simulink model "Demo_veDYNA_cs"  (Simulink 7.6)
settings: Solver=ode1  StartTime=0  StopTime=15  FixedStep=1/500  RelTol=1e-3
PreLoadFcn:
  | PreScanveDYNAPreLoadFcn(bdroot);
  | check_NUTS_defined;
  | 
  | assignin('base',['model_closed_' bdroot],false);
PostLoadFcn:
  | PreScanveDYNAPostLoadFcn(bdroot);
  | 
InitFcn:
  | vdy_SetExternalInputSource('ManLongCtrl',1,'Brake','other');
  | vdy_SetExternalInputSource('ManLongCtrl',1,'EngineTorque','other');
  | vdy_SetExternalInputSource('ManLatCtrl',1,'Steering','other');
  | 
  | PreScanveDYNAInitFcn(bdroot);
  | PreScanExperimentInitFcn(bdroot)
StopFcn:
  | PreScanExperimentStopFcn(bdroot)
undefined symbols (not defined in the file): at_period, CPT, vm_at_pulsewidth, vm_driver_dflt_gain, x_ini_VRML, y_ini_VRML, z_ini_VRML
libraries: dyna_cpt_lib x93, simulink x16, simulink_extras x14, PreScanSimulinkLibrary x6, anilib x3, dyna_lib x3, dyna_manctrl_lib x2, dyna_road_lib x2, PreScanUsefulBlocks x1, dyna_io_lib x1, dyna_demo_lib x1, dyna_usr_maneuver_states_lib x1
(part 5 of 8)

== system Demo_veDYNA_cs/Mazda_RX8_1/Simple ACC/Engine Torque Control/Demux Vehicle Info ==
  Vehicle Info : Inport
  vSoll : Inport  Port=2
  Bus Selector : BusSelector  OutputSignals=EngineTorqueMax[Nm],EngineTorqueMin[Nm],VehicleSpeed[m|s],TyreRadiusStatFront[m],GearRatioFront[],TyreRadiusStatRear[m],GearRatioRear[],VehicleMass[kg],EngineInertia[kgm2]
  gear_ratio : Subsystem
  mmot diff : Subsystem
  theta_red : Subsystem
  mmot_MAX : Outport
  mmot_MIN : Outport  Port=2
  v_akt1 : Outport  Port=3
  mmot_diff : Outport  Port=4
  wires:
  vSoll/1 -> mmot diff/5(vSoll)
  mmot diff/1(Out1) -> mmot_diff/1
  Bus Selector/2 -> mmot_MIN/1  "<EngineTorqueMin[Nm]>"
  Bus Selector/1 -> mmot_MAX/1  "<EngineTorqueMax[Nm]>"
  Bus Selector/3 -> v_akt1/1, mmot diff/1(vIst)  "<VehicleSpeed[m|s]>"
  theta_red/1(Theta) -> mmot diff/3(Theta)
  gear_ratio/1(GearRatio) -> theta_red/1(gear ratio), mmot diff/2(gear_ratio)
  Vehicle Info/1 -> Bus Selector/1
  Bus Selector/4 -> gear_ratio/1(RStatF)  "<TyreRadiusStatFront[m]>"
  Bus Selector/5 -> gear_ratio/2(GearRatioF)  "<GearRatioFront[]>"
  Bus Selector/6 -> gear_ratio/3(RStatR)  "<TyreRadiusStatRear[m]>"
  Bus Selector/7 -> gear_ratio/4(GearRatioR)  "<GearRatioRear[]>"
  Bus Selector/8 -> theta_red/2(VehMass)  "<VehicleMass[kg]>"
  Bus Selector/9 -> mmot diff/4(Theta Mot)  "<EngineInertia[kgm2]>"

== system Demo_veDYNA_cs/Mazda_RX8_1/Simple ACC/Engine Torque Control/Distance Control ==
  mmot_MAX : Inport
  mmot_MIN : Inport  Port=2
  v_akt : Inport  Port=3
  s_diff : Inport  Port=4
  Constant1 : Constant  Value=0
  Data Type Conversion1 : DataTypeConversion  SaturateOnIntegerOverflow=on  RndMeth=Zero
  Gain3 : Gain  Gain=-.1  SaturateOnIntegerOverflow=on  OutDataTypeStr=Inherit: Same as input  ParamDataTypeStr=Inherit: Same as input
  MinMax1 : MinMax  Function=max  Inputs=2  SaturateOnIntegerOverflow=on  InputSameDT=on
  MinMax2 : MinMax  Inputs=2  SaturateOnIntegerOverflow=on  InputSameDT=on
  P-Controller : Gain  Gain=6
  Product1 : Product  SaturateOnIntegerOverflow=on  InputSameDT=on  OutDataTypeStr=Inherit: Same as first input
  Relational Operator1 : RelationalOperator  Operator=>  InputSameDT=on
  Saturation1 : Saturate  UpperLimit=100  LowerLimit=0
  Sum : Sum  Inputs=|+-  SaturateOnIntegerOverflow=on  InputSameDT=on  OutDataTypeStr=Inherit: Same as first input
  dist_ratio : Gain  Gain=1.2  SaturateOnIntegerOverflow=on  OutDataTypeStr=Inherit: Same as input  ParamDataTypeStr=Inherit: Same as input
  Engine Torque : Outport
  Brake Pedal : Outport  Port=2
  wires:
  Saturation1/1 -> Brake Pedal/1
  Product1/1 -> Saturation1/1
  Gain3/1 -> Product1/2
  Data Type Conversion1/1 -> Product1/1
  Relational Operator1/1 -> Data Type Conversion1/1
  Constant1/1 -> Relational Operator1/1
  P-Controller/1 -> Gain3/1, Relational Operator1/2, MinMax1/1
  MinMax2/1 -> Engine Torque/1
  MinMax1/1 -> MinMax2/2
  mmot_MAX/1 -> MinMax2/1
  mmot_MIN/1 -> MinMax1/2
  dist_ratio/1 -> Sum/2
  Sum/1 -> P-Controller/1
  v_akt/1 -> dist_ratio/1
  s_diff/1 -> Sum/1

== system Demo_veDYNA_cs/Mazda_RX8_1/Simple ACC/Engine Torque Control/Speed Control ==
  mmot_MAX : Inport
  mmot_MIN : Inport  Port=2
  mmot_diff : Inport  Port=3
  MinMax : MinMax  Function=max  Inputs=2  SaturateOnIntegerOverflow=on  InputSameDT=on
  MinMax1 : MinMax  Inputs=2  SaturateOnIntegerOverflow=on  InputSameDT=on
  P-Controller : Gain  Gain=6
  Engine Torque : Outport
  wires:
  mmot_MIN/1 -> MinMax/2
  mmot_MAX/1 -> MinMax1/1
  MinMax1/1 -> Engine Torque/1
  MinMax/1 -> MinMax1/2
  P-Controller/1 -> MinMax/1
  mmot_diff/1 -> P-Controller/1

== system Demo_veDYNA_cs/Nissan_Cabstar_1/SELF_Demux/compas converter/cart2compas ==
  Angle [deg] : Inport
  Constant : Constant  Value=90
  Constant1 : Constant  Value=360
  Gain : Gain  Gain=1/360
  Gain1 : Gain  Gain=360
  Gain2 : Gain  Gain=-1
  Rounding Function : Rounding
  Sum : Sum  Inputs=|-+
  Sum1 : Sum  Inputs=-+|
  Sum2 : Sum  Inputs=++|
  heading [deg] : Outport
  wires:
  Sum2/1 -> heading [deg]/1
  Constant1/1 -> Sum2/1
  Gain2/1 -> Sum2/2
  Constant/1 -> Sum1/1
  Sum1/1 -> Sum/2, Gain/1
  Sum/1 -> Gain2/1
  Angle [deg]/1 -> Sum1/2
  Gain1/1 -> Sum/1
  Rounding Function/1 -> Gain1/1
  Gain/1 -> Rounding Function/1

== system Demo_veDYNA_cs/Nissan_Cabstar_1/Trajectories/Traj2State1/Traj2State2 ==
  traj : Inport
  MuxState : Subsystem
  Traj2MuxState_Ext : Subsystem
  state : Outport
  wires:
  Traj2MuxState_Ext/9(Y [rad]) -> MuxState/9(Y [rad])
  Traj2MuxState_Ext/8(P [rad]) -> MuxState/8(P [rad])
  Traj2MuxState_Ext/7(R [rad]) -> MuxState/7(R [rad])
  Traj2MuxState_Ext/6(dz [m/s]) -> MuxState/6(dz [m/s])
  Traj2MuxState_Ext/5(dy [m/s]) -> MuxState/5(dy [m/s])
  Traj2MuxState_Ext/4(dx [m/s]) -> MuxState/4(dx [m/s])
  Traj2MuxState_Ext/3(z [m]) -> MuxState/3(z [m])
  Traj2MuxState_Ext/2(y [m]) -> MuxState/2(y [m])
  Traj2MuxState_Ext/1(x [m]) -> MuxState/1(x [m])
  MuxState/1(state) -> state/1
  traj/1 -> Traj2MuxState_Ext/1(Traj)

== system Demo_veDYNA_cs/STATE_BMW_X5_1/state2FullState/limit roll/Substitute 90 & 270 deg (and its plurals) ==
  Angle [rad] : Inport
  270 deg detection : simulink/Model Verification/Check  Static Gap  Description=u <= 269.5 || 270.5 <= u  SystemSampleTime=-1  max=270.5  max_included=on  min=269.5  min_included=on  enabled=on  stopWhenAssertionFail=off  export=on  icon=graphic
  90 deg detection : simulink/Model Verification/Check  Static Gap  Description=u <= 89.5 || 90.5 <= u  SystemSampleTime=-1  max=90.5  max_included=on  min=89.5  min_included=on  enabled=on  stopWhenAssertionFail=off  export=on  icon=graphic
  Angle 0-360 deg limiter : Subsystem
  Degrees to Radians : simulink_extras/Transformations/Degrees to Radians  SystemSampleTime=-1
  Radians to Degrees : simulink_extras/Transformations/Radians to Degrees  SystemSampleTime=-1
  Substitution  Value : Constant  Value=269.5
  Substitution Value : Constant  Value=89.5
  Switch : Switch  Threshold=0.5
  Switch1 : Switch  Threshold=0.5
  Subst Angle [rad] : Outport
  wires:
  Angle [rad]/1 -> Radians to Degrees/1
  Degrees to Radians/1 -> Subst Angle [rad]/1
  Radians to Degrees/1 -> Angle 0-360 deg limiter/1(Angle [deg])
  Switch1/1 -> Degrees to Radians/1
  Substitution  Value/1 -> Switch1/3
  270 deg detection/1 -> Switch1/2
  Switch/1 -> Switch1/1, 270 deg detection/1
  Substitution Value/1 -> Switch/3
  90 deg detection/1 -> Switch/2
  Angle 0-360 deg limiter/1(LimAngle [deg]) -> 90 deg detection/1, Switch/1

== system Demo_veDYNA_cs/STATE_Mazda_RX8_1/state2FullState/limit roll/Substitute 90 & 270 deg (and its plurals) ==
  Angle [rad] : Inport
  270 deg detection : simulink/Model Verification/Check  Static Gap  Description=u <= 269.5 || 270.5 <= u  SystemSampleTime=-1  max=270.5  max_included=on  min=269.5  min_included=on  enabled=on  stopWhenAssertionFail=off  export=on  icon=graphic
  90 deg detection : simulink/Model Verification/Check  Static Gap  Description=u <= 89.5 || 90.5 <= u  SystemSampleTime=-1  max=90.5  max_included=on  min=89.5  min_included=on  enabled=on  stopWhenAssertionFail=off  export=on  icon=graphic
  Angle 0-360 deg limiter : Subsystem
  Degrees to Radians : simulink_extras/Transformations/Degrees to Radians  SystemSampleTime=-1
  Radians to Degrees : simulink_extras/Transformations/Radians to Degrees  SystemSampleTime=-1
  Substitution  Value : Constant  Value=269.5
  Substitution Value : Constant  Value=89.5
  Switch : Switch  Threshold=0.5
  Switch1 : Switch  Threshold=0.5
  Subst Angle [rad] : Outport
  wires:
  Angle [rad]/1 -> Radians to Degrees/1
  Degrees to Radians/1 -> Subst Angle [rad]/1
  Radians to Degrees/1 -> Angle 0-360 deg limiter/1(Angle [deg])
  Switch1/1 -> Degrees to Radians/1
  Substitution  Value/1 -> Switch1/3
  270 deg detection/1 -> Switch1/2
  Switch/1 -> Switch1/1, 270 deg detection/1
  Substitution Value/1 -> Switch/3
  90 deg detection/1 -> Switch/2
  Angle 0-360 deg limiter/1(LimAngle [deg]) -> 90 deg detection/1, Switch/1

== system Demo_veDYNA_cs/STATE_Nissan_Cabstar_1/state2FullState/limit roll/Substitute 90 & 270 deg (and its plurals) ==
  Angle [rad] : Inport
  270 deg detection : simulink/Model Verification/Check  Static Gap  Description=u <= 269.5 || 270.5 <= u  SystemSampleTime=-1  max=270.5  max_included=on  min=269.5  min_included=on  enabled=on  stopWhenAssertionFail=off  export=on  icon=graphic
  90 deg detection : simulink/Model Verification/Check  Static Gap  Description=u <= 89.5 || 90.5 <= u  SystemSampleTime=-1  max=90.5  max_included=on  min=89.5  min_included=on  enabled=on  stopWhenAssertionFail=off  export=on  icon=graphic
  Angle 0-360 deg limiter : Subsystem
  Degrees to Radians : simulink_extras/Transformations/Degrees to Radians  SystemSampleTime=-1
  Radians to Degrees : simulink_extras/Transformations/Radians to Degrees  SystemSampleTime=-1
  Substitution  Value : Constant  Value=269.5
  Substitution Value : Constant  Value=89.5
  Switch : Switch  Threshold=0.5
  Switch1 : Switch  Threshold=0.5
  Subst Angle [rad] : Outport
  wires:
  Angle [rad]/1 -> Radians to Degrees/1
  Degrees to Radians/1 -> Subst Angle [rad]/1
  Radians to Degrees/1 -> Angle 0-360 deg limiter/1(Angle [deg])
  Switch1/1 -> Degrees to Radians/1
  Substitution  Value/1 -> Switch1/3
  270 deg detection/1 -> Switch1/2
  Switch/1 -> Switch1/1, 270 deg detection/1
  Substitution Value/1 -> Switch/3
  90 deg detection/1 -> Switch/2
  Angle 0-360 deg limiter/1(LimAngle [deg]) -> 90 deg detection/1, Switch/1

== system Demo_veDYNA_cs/Vedyna_Vehicle/CPT_MDL/MDL_PAR/BrkHyd ==
  System Instance 1 : Subsystem
      mask Display: disp('[Generated]')

== system Demo_veDYNA_cs/Vedyna_Vehicle/CPT_MDL/MDL_PAR/ClutchCtrl ==
  System Instance 1 : Subsystem
      mask Display: disp('[Generated]')

== system Demo_veDYNA_cs/Vedyna_Vehicle/CPT_MDL/MDL_PAR/Contact ==
  System Instance 1 : Subsystem
      mask Display: disp('[Generated]')
  System Instance 2 : Subsystem
      mask Display: disp('[Generated]')
  System Instance 3 : Subsystem
      mask Display: disp('[Generated]')
  System Instance 4 : Subsystem
      mask Display: disp('[Generated]')
  System Instance 5 : Subsystem
      mask Display: disp('[Generated]')
  System Instance 6 : Subsystem
      mask Display: disp('[Generated]')
  System Instance 7 : Subsystem
      mask Display: disp('[Generated]')
  System Instance 8 : Subsystem
      mask Display: disp('[Generated]')

== system Demo_veDYNA_cs/Vedyna_Vehicle/CPT_MDL/MDL_PAR/Driver ==
  System Instance 1 : Subsystem
      mask Display: disp('[Generated]')

== system Demo_veDYNA_cs/Vedyna_Vehicle/CPT_MDL/MDL_PAR/Engine ==
  System Instance 1 : Subsystem
      mask Display: disp('[Generated]')

== system Demo_veDYNA_cs/Vedyna_Vehicle/CPT_MDL/MDL_PAR/GearCtrl ==
  System Instance 1 : Subsystem
      mask Display: disp('[Generated]')

== system Demo_veDYNA_cs/Vedyna_Vehicle/CPT_MDL/MDL_PAR/ManLatCtrl ==
  System Instance 1 : Subsystem
      mask Display: disp('[Generated]')

== system Demo_veDYNA_cs/Vedyna_Vehicle/CPT_MDL/MDL_PAR/ManLongCtrl ==
  System Instance 1 : Subsystem
      mask Display: disp('[Generated]')

== system Demo_veDYNA_cs/Vedyna_Vehicle/CPT_MDL/MDL_PAR/ManSchedule ==

== system Demo_veDYNA_cs/Vedyna_Vehicle/CPT_MDL/MDL_PAR/Tmeasy ==
  System Instance 1 : Subsystem
      mask Display: disp('[Generated]')
  System Instance 2 : Subsystem
      mask Display: disp('[Generated]')
  System Instance 3 : Subsystem
      mask Display: disp('[Generated]')
  System Instance 4 : Subsystem
      mask Display: disp('[Generated]')
  System Instance 5 : Subsystem
      mask Display: disp('[Generated]')
  System Instance 6 : Subsystem
      mask Display: disp('[Generated]')
  System Instance 7 : Subsystem
      mask Display: disp('[Generated]')
  System Instance 8 : Subsystem
      mask Display: disp('[Generated]')

== system Demo_veDYNA_cs/Vedyna_Vehicle/CPT_MDL/MDL_PAR/Wheel ==
  System Instance 1 : Subsystem
      mask Display: disp('[Generated]')
  System Instance 2 : Subsystem
      mask Display: disp('[Generated]')
  System Instance 3 : Subsystem
      mask Display: disp('[Generated]')
  System Instance 4 : Subsystem
      mask Display: disp('[Generated]')
  System Instance 5 : Subsystem
      mask Display: disp('[Generated]')
  System Instance 6 : Subsystem
      mask Display: disp('[Generated]')
  System Instance 7 : Subsystem
      mask Display: disp('[Generated]')
  System Instance 8 : Subsystem
      mask Display: disp('[Generated]')

== system Demo_veDYNA_cs/Vedyna_Vehicle/CPT_MDL/MDL_SW/BrkHyd ==
  System Instance 1 : Subsystem
      mask Display: disp('[Generated]')

== system Demo_veDYNA_cs/Vedyna_Vehicle/CPT_MDL/MDL_SW/Chassis ==
  System Instance 1 : Subsystem
      mask Display: disp('[Generated]')

== system Demo_veDYNA_cs/Vedyna_Vehicle/CPT_MDL/MDL_SW/ClutchCtrl ==
  System Instance 1 : Subsystem
      mask Display: disp('[Generated]')

== system Demo_veDYNA_cs/Vedyna_Vehicle/CPT_MDL/MDL_SW/Contact ==
  System Instance 1 : Subsystem
      mask Display: disp('[Generated]')
  System Instance 2 : Subsystem
      mask Display: disp('[Generated]')
  System Instance 3 : Subsystem
      mask Display: disp('[Generated]')
  System Instance 4 : Subsystem
      mask Display: disp('[Generated]')
  System Instance 5 : Subsystem
      mask Display: disp('[Generated]')
  System Instance 6 : Subsystem
      mask Display: disp('[Generated]')
  System Instance 7 : Subsystem
      mask Display: disp('[Generated]')
  System Instance 8 : Subsystem
      mask Display: disp('[Generated]')

== system Demo_veDYNA_cs/Vedyna_Vehicle/CPT_MDL/MDL_SW/Driveline ==
  System Instance 1 : Subsystem
      mask Display: disp('[Generated]')

== system Demo_veDYNA_cs/Vedyna_Vehicle/CPT_MDL/MDL_SW/Driver ==
  System Instance 1 : Subsystem
      mask Display: disp('[Generated]')

== system Demo_veDYNA_cs/Vedyna_Vehicle/CPT_MDL/MDL_SW/Engine ==
  System Instance 1 : Subsystem
      mask Display: disp('[Generated]')

== system Demo_veDYNA_cs/Vedyna_Vehicle/CPT_MDL/MDL_SW/GearCtrl ==
  System Instance 1 : Subsystem
      mask Display: disp('[Generated]')

== system Demo_veDYNA_cs/Vedyna_Vehicle/CPT_MDL/MDL_SW/ManLatCtrl ==
  System Instance 1 : Subsystem
      mask Display: disp('[Generated]')

== system Demo_veDYNA_cs/Vedyna_Vehicle/CPT_MDL/MDL_SW/ManLongCtrl ==
  System Instance 1 : Subsystem
      mask Display: disp('[Generated]')

== system Demo_veDYNA_cs/Vedyna_Vehicle/CPT_MDL/MDL_SW/ManSchedule ==
  System Instance 1 : Subsystem
      mask Display: disp('[Generated]')
  System Instance 2 : Subsystem
      mask Display: disp('[Generated]')
  System Instance 3 : Subsystem
      mask Display: disp('[Generated]')

== system Demo_veDYNA_cs/Vedyna_Vehicle/CPT_MDL/MDL_SW/Road ==
  System Instance 1 : Subsystem
      mask Display: disp('[Generated]')

== system Demo_veDYNA_cs/Vedyna_Vehicle/CPT_MDL/MDL_SW/Simctrl ==
  System Instance 1 : Subsystem
      mask Display: disp('[Generated]')

== system Demo_veDYNA_cs/Vedyna_Vehicle/CPT_MDL/MDL_SW/Tmeasy ==
  System Instance 1 : Subsystem
      mask Display: disp('[Generated]')
  System Instance 2 : Subsystem
      mask Display: disp('[Generated]')
  System Instance 3 : Subsystem
      mask Display: disp('[Generated]')
  System Instance 4 : Subsystem
      mask Display: disp('[Generated]')
  System Instance 5 : Subsystem
      mask Display: disp('[Generated]')
  System Instance 6 : Subsystem
      mask Display: disp('[Generated]')
  System Instance 7 : Subsystem
      mask Display: disp('[Generated]')
  System Instance 8 : Subsystem
      mask Display: disp('[Generated]')

== system Demo_veDYNA_cs/Vedyna_Vehicle/CPT_MDL/MDL_SW/Vehicle ==
  System Instance 1 : Subsystem
      mask Display: disp('[Generated]')

== system Demo_veDYNA_cs/Vedyna_Vehicle/CPT_MDL/MDL_SW/Wheel ==
  System Instance 1 : Subsystem
      mask Display: disp('[Generated]')
  System Instance 2 : Subsystem
      mask Display: disp('[Generated]')
  System Instance 3 : Subsystem
      mask Display: disp('[Generated]')
  System Instance 4 : Subsystem
      mask Display: disp('[Generated]')
  System Instance 5 : Subsystem
      mask Display: disp('[Generated]')
  System Instance 6 : Subsystem
      mask Display: disp('[Generated]')
  System Instance 7 : Subsystem
      mask Display: disp('[Generated]')
  System Instance 8 : Subsystem
      mask Display: disp('[Generated]')

== system Demo_veDYNA_cs/Vedyna_Vehicle/vdy_mdl/Maneuver Control/HCI Switch Driver ==
  Mux3 : Mux  Inputs=3
  SW_ClutchCtrl_1_HCI : dyna_cpt_lib/CPT_MDL_HCI_SW_ACCESS  Tag=vedynaCPT_MDL_HCI_SW_ACCESS  component=ClutchCtrl  system_inst=1  parameter=HCI
  SW_Driver_1_HCI : dyna_cpt_lib/CPT_MDL_HCI_SW_ACCESS  Tag=vedynaCPT_MDL_HCI_SW_ACCESS  component=Driver  system_inst=1  parameter=HCI
  SW_GearCtrl_1_HCI : dyna_cpt_lib/CPT_MDL_HCI_SW_ACCESS  Tag=vedynaCPT_MDL_HCI_SW_ACCESS  component=GearCtrl  system_inst=1  parameter=HCI
  HCI manCtrl : Outport
  wires:
  Mux3/1 -> HCI manCtrl/1
  SW_ClutchCtrl_1_HCI/1 -> Mux3/3
  SW_GearCtrl_1_HCI/1 -> Mux3/2
  SW_Driver_1_HCI/1 -> Mux3/1

== system Demo_veDYNA_cs/Vedyna_Vehicle/vdy_mdl/Maneuver Control/HCI Switches ==
  Mux : Mux  Inputs=3
  SW_ManSchedule_1_HCI : dyna_cpt_lib/CPT_MDL_HCI_SW_ACCESS  Tag=vedynaCPT_MDL_HCI_SW_ACCESS  component=ManSchedule  system_inst=1  parameter=HCI
  SW_ManSchedule_2_HCI : dyna_cpt_lib/CPT_MDL_HCI_SW_ACCESS  Tag=vedynaCPT_MDL_HCI_SW_ACCESS  component=ManSchedule  system_inst=2  parameter=HCI
  SW_ManSchedule_3_HCI : dyna_cpt_lib/CPT_MDL_HCI_SW_ACCESS  Tag=vedynaCPT_MDL_HCI_SW_ACCESS  component=ManSchedule  system_inst=3  parameter=HCI
  "HCI Switches " : Outport
  wires:
  SW_ManSchedule_3_HCI/1 -> Mux/3
  SW_ManSchedule_2_HCI/1 -> Mux/2
  SW_ManSchedule_1_HCI/1 -> Mux/1
  Mux/1 -> "HCI Switches "/1

== system Demo_veDYNA_cs/Vedyna_Vehicle/vdy_mdl/Maneuver Control/Maneuver Controller Inputs ==
  Clutch Control Inputs : Subsystem
  Driver Inputs : Subsystem
  Gear Control Inputs : Subsystem
  Lateral Control Inputs : Subsystem
  Longitudinal Control Inputs : Subsystem
  "Longitudinal Control Inputs " : Outport
  "Lateral Control Inputs " : Outport  Port=2
  "Driver Inputs " : Outport  Port=3
  "Gear Control Inputs " : Outport  Port=4
  "Clutch Control Inputs " : Outport  Port=5
  wires:
  Driver Inputs/1(Driver Inputs) -> "Driver Inputs "/1
  Gear Control Inputs/1(Gear Control Inputs) -> "Gear Control Inputs "/1
  Clutch Control Inputs/1(Clutch Control Inputs) -> "Clutch Control Inputs "/1
  Lateral Control Inputs/1(Lateral Control Inputs) -> "Lateral Control Inputs "/1
  Longitudinal Control Inputs/1(Longitudinal Control Inputs) -> "Longitudinal Control Inputs "/1

== system Demo_veDYNA_cs/Vedyna_Vehicle/vdy_mdl/Maneuver Control/Maneuver Scheduler Inputs ==
  Vehicle Info : Inport
  Demux : Demux  Outputs=[2,-1]
  Demux1 : Demux  Outputs=[3 1 1 1 1]
  Dot Product : DotProduct  InputSameDT=on  OutDataTypeStr=Inherit: Inherit via internal rule
  Math Functio : Math  Operator=sqrt  SaturateOnIntegerOverflow=on
  Mux1 : Mux  Inputs=3
  Mux2 : Mux  Inputs=6
  Road Information : dyna_road_lib/Road Information  comp_name=Road  RdQueryTyp=xy  nq=1  rd_info_lib=vm_road_info_lib
  Selector4 : Selector  InputPortWidth=21  IndexOptions=Index vector (dialog)  Indices=[1]  OutputSizes=1
  User Definition of Maneuver End States : dyna_usr_maneuver_states_lib/User Definition of Maneuver End States
  m/s_km/h : Gain  Gain=3.6  SaturateOnIntegerOverflow=on  OutDataTypeStr=Inherit: Same as input  ParamDataTypeStr=Inherit: Same as input
  rad_deg : Gain  Gain=180/pi  SaturateOnIntegerOverflow=on  OutDataTypeStr=Inherit: Same as input  ParamDataTypeStr=Inherit: Same as input
  rad_deg1 : Gain  Gain=1e-5  SaturateOnIntegerOverflow=on  OutDataTypeStr=Inherit: Same as input  ParamDataTypeStr=Inherit: Same as input
  rad_deg2 : Gain  Gain=180/pi  SaturateOnIntegerOverflow=on  OutDataTypeStr=Inherit: Same as input  ParamDataTypeStr=Inherit: Same as input
  state_from_vehicleinfo : Selector  IndexOptions=Index vector (dialog)  Indices=[7,8,10,11,12,38,14,66,65]  OutputSizes=1
  Control States : Outport
  wires:
  Demux1/1 -> Dot Product/2, Dot Product/1  "velocity[m/s]"
  Math Functio/1 -> m/s_km/h/1
  Dot Product/1 -> Math Functio/1
  User Definition of Maneuver End States/1 -> Mux2/6
  Mux2/1 -> Mux1/3
  Demux/2 -> Demux1/1
  rad_deg2/1 -> Mux2/5  "[deg/s]"
  rad_deg1/1 -> Mux2/4  "[bar]"
  rad_deg/1 -> Mux2/2  "[deg]"
  m/s_km/h/1 -> Mux2/1  "[km/h]"
  Demux1/5 -> rad_deg2/1  "roll rate [rad/s]"
  Demux1/2 -> rad_deg/1  "steering wheel angle [rad]"
  Demux1/3 -> Mux2/3  "lateral acc.[m/s**2]"
  Demux1/4 -> rad_deg1/1  "brake pressure [Pa]"
  state_from_vehicleinfo/1 -> Demux/1
  Demux/1 -> Road Information/1
  Selector4/1 -> Mux1/2  "distance [m]"
  Mux1/1 -> Control States/1
  [vdy_Simctrl_tsim] -> Mux1/1  "Simulation time [s]"
  Road Information/1 -> Selector4/1
  Vehicle Info/1 -> state_from_vehicleinfo/1

== system Demo_veDYNA_cs/Vedyna_Vehicle/vdy_mdl/Road/veDYNA Road Subsystem ==
  note: veDYNA Road Subsystem
  note: COPYRIGHT 2002 by TESIS DYNAware GmbH
  SyncIn : Inport
  HCI Switch : Subsystem
  veDYNA Road : dyna_road_lib/veDYNA Road
  SyncOut : Outport
  wires:
  HCI Switch/1(HCI Switch) -> veDYNA Road/2
  veDYNA Road/1 -> SyncOut/1
  SyncIn/1 -> veDYNA Road/1

== system Demo_veDYNA_cs/Vedyna_Vehicle/vdy_mdl/Simulation Control/veDYNA Simulation Control Subsystem ==
  note: veDYNA Simulation Control Subsystem
  note: COPYRIGHT 2002 by TESIS DYNAware GmbH
  SyncIn : Inport
  SW_Simctrl_1_Reset : dyna_cpt_lib/CPT_MDL_SW_ACCESS  Tag=vedynaCPT_MDL_HCI_ACCESS  component=Simctrl  system_inst=1  parameter=Reset
  veDYNA Simulation Control : dyna_simctrl_lib/veDYNA Simulation Control  Tag=vedynaSimctrlMask
  SyncOut : Outport
  wires:
  SW_Simctrl_1_Reset/1 -> veDYNA Simulation Control/2
  veDYNA Simulation Control/1 -> SyncOut/1
  SyncIn/1 -> veDYNA Simulation Control/1

== system Demo_veDYNA_cs/Vedyna_Vehicle/vdy_mdl/Vehicle System/veDYNA Vehicle Subsystem ==
  note: veDYNA Vehicle Subsystem
  note: COPYRIGHT 2002 by TESIS DYNAware GmbH
  SyncIn : Inport
  Maneuver Commands : Inport  Port=2
  Input from I/O : Inport  Port=3
  External Body Forces : Inport  Port=4
  Brake System : Subsystem
  External Vehicle Inputs (from I/O) : Subsystem
  HCI Switches : Subsystem
  Maneuver Commands Splitter : Subsystem
  Mux : Mux  Inputs=2
  Selector : Selector  InputPortWidth=32  IndexOptions=Index vector (dialog)  Indices=[1:4]  OutputSizes=1
  Selector1 : Selector  InputPortWidth=32  IndexOptions=Index vector (dialog)  Indices=[5:18]  OutputSizes=1
  Vehicle Outputs to I/O : Subsystem
  veDYNA Vehicle : dyna_vehicle_lib/veDYNA Vehicle
  Output to I/O : Outport
  Vehicle Info : Outport  Port=2
  Reference System : Outport  Port=3
  SyncOut : Outport  Port=4
  wires:
  HCI Switches/1(HCI Switches) -> veDYNA Vehicle/7
  Selector1/1 -> Brake System/2(I/O Vector)
  Selector/1 -> External Vehicle Inputs (from I/O)/2(I/O Vector)
  Input from I/O/1 -> Selector/1, Selector1/1
  Mux/1 -> Vehicle Info/1
  Vehicle Outputs to I/O/2(SyncOut) -> SyncOut/1
  Vehicle Outputs to I/O/1(Output to IO) -> Output to I/O/1
  veDYNA Vehicle/3 -> Vehicle Outputs to I/O/1(SyncIn)
  External Vehicle Inputs (from I/O)/2(External Inputs) -> veDYNA Vehicle/5
  External Body Forces/1 -> veDYNA Vehicle/6
  External Vehicle Inputs (from I/O)/1(SyncOut) -> Brake System/1(SyncIn)
  veDYNA Vehicle/1 -> Mux/2
  Brake System/1(Brake Hydraulics Info) -> Mux/1
  Brake System/2(SyncOut) -> veDYNA Vehicle/1
  Brake System/3(Master Cylinder Pressure) -> veDYNA Vehicle/2
  Brake System/4(Wheel Cylinder Pressures) -> veDYNA Vehicle/3
  veDYNA Vehicle/2 -> Reference System/1
  Maneuver Commands Splitter/4(Maneuver Commands to Vehicle) -> veDYNA Vehicle/4
  Maneuver Commands/1 -> Maneuver Commands Splitter/2(Maneuver Commands)
  SyncIn/1 -> Maneuver Commands Splitter/1(SyncIn)
  Maneuver Commands Splitter/3(Maneuver Commands to Brake System) -> Brake System/3(Brake Pedal Position)
  Maneuver Commands Splitter/2(Maneuver Commands to External Inputs) -> External Vehicle Inputs (from I/O)/3(Maneuver Commands)
  Maneuver Commands Splitter/1(SyncOut) -> External Vehicle Inputs (from I/O)/1(SyncIn)

== system Demo_veDYNA_cs/BMW_X5_1/Trajectories/Traj2State1/Traj2State2/MuxState ==
  x [m] : Inport
  y [m] : Inport  Port=2
  z [m] : Inport  Port=3
  dx [m/s] : Inport  Port=4
  dy [m/s] : Inport  Port=5
  dz [m/s] : Inport  Port=6
  R [rad] : Inport  Port=7
  P [rad] : Inport  Port=8
  Y [rad] : Inport  Port=9
  Mux : Mux  Inputs=9
  state : Outport
  wires:
  z [m]/1 -> Mux/3
  y [m]/1 -> Mux/2
  x [m]/1 -> Mux/1
  Y [rad]/1 -> Mux/9
  P [rad]/1 -> Mux/8
  R [rad]/1 -> Mux/7
  dz [m/s]/1 -> Mux/6
  dy [m/s]/1 -> Mux/5
  dx [m/s]/1 -> Mux/4
  Mux/1 -> state/1

== system Demo_veDYNA_cs/BMW_X5_1/Trajectories/Traj2State1/Traj2State2/Traj2MuxState_Ext ==
  Traj : Inport
  Terminator{1..9} (9 alike) : Terminator
  demux : Subsystem
  x [m] : Outport
  y [m] : Outport  Port=2
  z [m] : Outport  Port=3
  dx [m/s] : Outport  Port=4
  dy [m/s] : Outport  Port=5
  dz [m/s] : Outport  Port=6
  R [rad] : Outport  Port=7
  P [rad] : Outport  Port=8
  Y [rad] : Outport  Port=9
  wires:
  demux/9(Y) -> Y [rad]/1
  demux/7(R) -> R [rad]/1
  demux/5(vely) -> dy [m/s]/1
  demux/4(velx) -> dx [m/s]/1
  demux/10(velR) -> Terminator4/1
  demux/11(velP) -> Terminator5/1
  demux/12(velY) -> Terminator1/1
  demux/13(accx) -> Terminator8/1
  demux/14(accy) -> Terminator9/1
  demux/15(accz) -> Terminator7/1
  demux/18(accY) -> Terminator2/1
  demux/16(accR) -> Terminator3/1
  demux/17(accP) -> Terminator6/1
  demux/3(z) -> z [m]/1
  Traj/1 -> demux/1(traj)
  demux/6(velz) -> dz [m/s]/1
  demux/1(x) -> x [m]/1
  demux/2(y) -> y [m]/1
  demux/8(P) -> P [rad]/1

== system Demo_veDYNA_cs/Mazda_RX8_1/Simple ACC/Engine Torque Control/Demux Vehicle Info/gear_ratio ==
  RStatF : Inport
  GearRatioF : Inport  Port=2
  RStatR : Inport  Port=3
  GearRatioR : Inport  Port=4
  Product1 : Product  Inputs=/*  SaturateOnIntegerOverflow=on  InputSameDT=on  OutDataTypeStr=Inherit: Same as first input
  Product2 : Product  Inputs=/*  SaturateOnIntegerOverflow=on  InputSameDT=on  OutDataTypeStr=Inherit: Same as first input
  Sum : Sum  Inputs=|++  SaturateOnIntegerOverflow=on  InputSameDT=on  OutDataTypeStr=Inherit: Same as first input
  GearRatio : Outport
  wires:
  Sum/1 -> GearRatio/1
  Product2/1 -> Sum/1
  Product1/1 -> Sum/2
  RStatF/1 -> Product2/1
  GearRatioF/1 -> Product2/2
  RStatR/1 -> Product1/1
  GearRatioR/1 -> Product1/2

== system Demo_veDYNA_cs/Mazda_RX8_1/Simple ACC/Engine Torque Control/Demux Vehicle Info/mmot diff ==
  vIst : Inport
  gear_ratio : Inport  Port=2
  Theta : Inport  Port=3
  Theta Mot : Inport  Port=4
  vSoll : Inport  Port=5
  Product : Product  Inputs=3  SaturateOnIntegerOverflow=on  InputSameDT=on  OutDataTypeStr=Inherit: Same as first input
  Sum : Sum  Inputs=|++  SaturateOnIntegerOverflow=on  InputSameDT=on  OutDataTypeStr=Inherit: Same as first input
  Sum1 : Sum  Inputs=+-  SaturateOnIntegerOverflow=on  InputSameDT=on  OutDataTypeStr=Inherit: Same as first input
  Out1 : Outport
  wires:
  Product/1 -> Out1/1
  Sum1/1 -> Product/1
  Sum/1 -> Product/3
  gear_ratio/1 -> Product/2
  vSoll/1 -> Sum1/1
  vIst/1 -> Sum1/2
  Theta/1 -> Sum/1
  Theta Mot/1 -> Sum/2

== system Demo_veDYNA_cs/Mazda_RX8_1/Simple ACC/Engine Torque Control/Demux Vehicle Info/theta_red ==
  gear ratio : Inport
  VehMass : Inport  Port=2
  Constant : Constant
  Math Function : Math  Operator=square  SaturateOnIntegerOverflow=on
  Product1 : Product  Inputs=/*  SaturateOnIntegerOverflow=on  InputSameDT=on  OutDataTypeStr=Inherit: Same as first input
  Sum : Sum  Inputs=++|  SaturateOnIntegerOverflow=on  InputSameDT=on  OutDataTypeStr=Inherit: Same as first input
  Theta : Outport
  wires:
  Constant/1 -> Sum/1
  Sum/1 -> Product1/1
  Math Function/1 -> Sum/2
  gear ratio/1 -> Math Function/1
  Product1/1 -> Theta/1
  VehMass/1 -> Product1/2

== system Demo_veDYNA_cs/Nissan_Cabstar_1/Trajectories/Traj2State1/Traj2State2/MuxState ==
  x [m] : Inport
  y [m] : Inport  Port=2
  z [m] : Inport  Port=3
  dx [m/s] : Inport  Port=4
  dy [m/s] : Inport  Port=5
  dz [m/s] : Inport  Port=6
  R [rad] : Inport  Port=7
  P [rad] : Inport  Port=8
  Y [rad] : Inport  Port=9
  Mux : Mux  Inputs=9
  state : Outport
  wires:
  z [m]/1 -> Mux/3
  y [m]/1 -> Mux/2
  x [m]/1 -> Mux/1
  Y [rad]/1 -> Mux/9
  P [rad]/1 -> Mux/8
  R [rad]/1 -> Mux/7
  dz [m/s]/1 -> Mux/6
  dy [m/s]/1 -> Mux/5
  dx [m/s]/1 -> Mux/4
  Mux/1 -> state/1

== system Demo_veDYNA_cs/Nissan_Cabstar_1/Trajectories/Traj2State1/Traj2State2/Traj2MuxState_Ext ==
  Traj : Inport
  Terminator{1..9} (9 alike) : Terminator
  demux : Subsystem
  x [m] : Outport
  y [m] : Outport  Port=2
  z [m] : Outport  Port=3
  dx [m/s] : Outport  Port=4
  dy [m/s] : Outport  Port=5
  dz [m/s] : Outport  Port=6
  R [rad] : Outport  Port=7
  P [rad] : Outport  Port=8
  Y [rad] : Outport  Port=9
  wires:
  demux/9(Y) -> Y [rad]/1
  demux/7(R) -> R [rad]/1
  demux/5(vely) -> dy [m/s]/1
  demux/4(velx) -> dx [m/s]/1
  demux/10(velR) -> Terminator4/1
  demux/11(velP) -> Terminator5/1
  demux/12(velY) -> Terminator1/1
  demux/13(accx) -> Terminator8/1
  demux/14(accy) -> Terminator9/1
  demux/15(accz) -> Terminator7/1
  demux/18(accY) -> Terminator2/1
  demux/16(accR) -> Terminator3/1
  demux/17(accP) -> Terminator6/1
  demux/3(z) -> z [m]/1
  Traj/1 -> demux/1(traj)
  demux/6(velz) -> dz [m/s]/1
  demux/1(x) -> x [m]/1
  demux/2(y) -> y [m]/1
  demux/8(P) -> P [rad]/1

== system Demo_veDYNA_cs/STATE_BMW_X5_1/state2FullState/limit roll/Substitute 90 & 270 deg (and its plurals)/Angle 0-360 deg limiter ==
  Angle [deg] : Inport
  Gain : Gain  Gain=1/360
  Gain1 : Gain  Gain=360
  Rounding Function : Rounding
  Sum : Sum  Inputs=|-+
  LimAngle [deg] : Outport
  wires:
  Gain/1 -> Rounding Function/1
  Rounding Function/1 -> Gain1/1
  Gain1/1 -> Sum/1
  Angle [deg]/1 -> Gain/1, Sum/2
  Sum/1 -> LimAngle [deg]/1

== system Demo_veDYNA_cs/STATE_Mazda_RX8_1/state2FullState/limit roll/Substitute 90 & 270 deg (and its plurals)/Angle 0-360 deg limiter ==
  Angle [deg] : Inport
  Gain : Gain  Gain=1/360
  Gain1 : Gain  Gain=360
  Rounding Function : Rounding
  Sum : Sum  Inputs=|-+
  LimAngle [deg] : Outport
  wires:
  Gain/1 -> Rounding Function/1
  Rounding Function/1 -> Gain1/1
  Gain1/1 -> Sum/1
  Angle [deg]/1 -> Gain/1, Sum/2
  Sum/1 -> LimAngle [deg]/1

== system Demo_veDYNA_cs/STATE_Nissan_Cabstar_1/state2FullState/limit roll/Substitute 90 & 270 deg (and its plurals)/Angle 0-360 deg limiter ==
  Angle [deg] : Inport
  Gain : Gain  Gain=1/360
  Gain1 : Gain  Gain=360
  Rounding Function : Rounding
  Sum : Sum  Inputs=|-+
  LimAngle [deg] : Outport
  wires:
  Gain/1 -> Rounding Function/1
  Rounding Function/1 -> Gain1/1
  Gain1/1 -> Sum/1
  Angle [deg]/1 -> Gain/1, Sum/2
  Sum/1 -> LimAngle [deg]/1

== system Demo_veDYNA_cs/Vedyna_Vehicle/CPT_MDL/MDL_PAR/BrkHyd/System Instance 1 ==
  pbrmaster [N/m**2] : Subsystem
      mask Display: disp('Master brake cylinder pressure [N/m**2]')

== system Demo_veDYNA_cs/Vedyna_Vehicle/CPT_MDL/MDL_PAR/ClutchCtrl/System Instance 1 ==
  Clutch [%] : Subsystem
      mask Display: disp('Clutch ratio [%]')

== system Demo_veDYNA_cs/Vedyna_Vehicle/CPT_MDL/MDL_PAR/Contact/System Instance 1 ==
  RoadZ [m] : Subsystem
      mask Display: disp('Local road excitation [m]')

== system Demo_veDYNA_cs/Vedyna_Vehicle/CPT_MDL/MDL_PAR/Contact/System Instance 2 ==
  RoadZ [m] : Subsystem
      mask Display: disp('Local road excitation [m]')

== system Demo_veDYNA_cs/Vedyna_Vehicle/CPT_MDL/MDL_PAR/Contact/System Instance 3 ==
  RoadZ [m] : Subsystem
      mask Display: disp('Local road excitation [m]')

== system Demo_veDYNA_cs/Vedyna_Vehicle/CPT_MDL/MDL_PAR/Contact/System Instance 4 ==
  RoadZ [m] : Subsystem
      mask Display: disp('Local road excitation [m]')

== system Demo_veDYNA_cs/Vedyna_Vehicle/CPT_MDL/MDL_PAR/Contact/System Instance 5 ==
  RoadZ [m] : Subsystem
      mask Display: disp('Local road excitation [m]')

== system Demo_veDYNA_cs/Vedyna_Vehicle/CPT_MDL/MDL_PAR/Contact/System Instance 6 ==
  RoadZ [m] : Subsystem
      mask Display: disp('Local road excitation [m]')

== system Demo_veDYNA_cs/Vedyna_Vehicle/CPT_MDL/MDL_PAR/Contact/System Instance 7 ==
  RoadZ [m] : Subsystem
      mask Display: disp('Local road excitation [m]')

== system Demo_veDYNA_cs/Vedyna_Vehicle/CPT_MDL/MDL_PAR/Contact/System Instance 8 ==
  RoadZ [m] : Subsystem
      mask Display: disp('Local road excitation [m]')

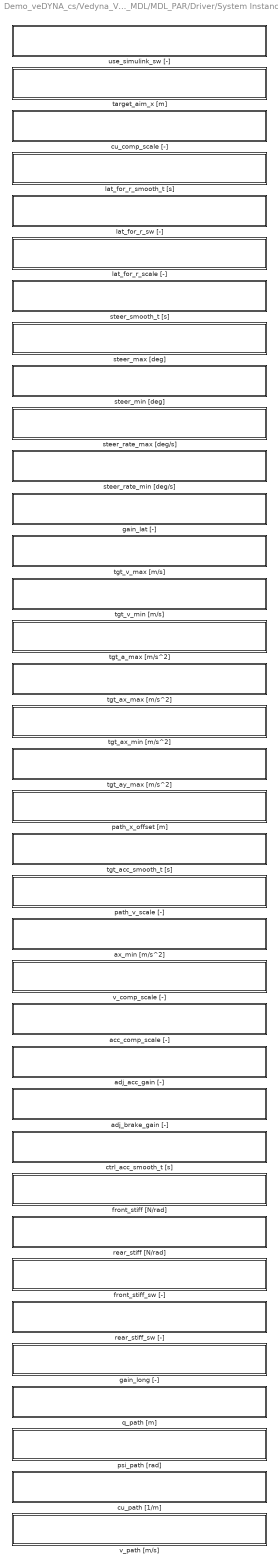
== system Demo_veDYNA_cs/Vedyna_Vehicle/CPT_MDL/MDL_PAR/Driver/System Instance 1 ==
  acc_comp_scale [-] : Subsystem
      mask Display: disp('v (acc_comp_scale) [-]')
  adj_acc_gain [-] : Subsystem
      mask Display: disp('v (adj_acc_gain) [-]')
  adj_brake_gain [-] : Subsystem
      mask Display: disp('v (adj_brake_gain) [-]')
  ax_min [m/s^2] : Subsystem
      mask Display: disp('v (ax_min) [m/s^2]')
  ctrl_acc_smooth_t [s] : Subsystem
      mask Display: disp('v (ctrl_acc_smooth_t) [s]')
  cu_comp_scale [-] : Subsystem
      mask Display: disp('v (cu_comp_scale) [-]')
  cu_path [1/m] : Subsystem
      mask Display: disp('path curvature [1/m]')
  front_stiff [N/rad] : Subsystem
      mask Display: disp('v (front_stiff) [N/rad]')
  front_stiff_sw [-] : Subsystem
      mask Display: disp('v (front_stiff_sw) [-]')
  gain_lat [-] : Subsystem
      mask Display: disp('v (gain_lat) [-]')
  gain_long [-] : Subsystem
      mask Display: disp('v (gain_long) [-]')
  lat_for_r_scale [-] : Subsystem
      mask Display: disp('v (lat_for_r_scale) [-]')
  lat_for_r_smooth_t [s] : Subsystem
      mask Display: disp('v (lat_for_r_smooth_t) [s]')
  lat_for_r_sw [-] : Subsystem
      mask Display: disp('v (lat_for_r_sw) [-]')
  path_v_scale [-] : Subsystem
      mask Display: disp('v (path_v_scale) [-]')
  path_x_offset [m] : Subsystem
      mask Display: disp('v (path_x_offset) [m]')
  psi_path [rad] : Subsystem
      mask Display: disp('path angle offset (relative to road''s center line) [rad]')
  q_path [m] : Subsystem
      mask Display: disp('lateral offset [m]')
  rear_stiff [N/rad] : Subsystem
      mask Display: disp('v (rear_stiff) [N/rad]')
  rear_stiff_sw [-] : Subsystem
      mask Display: disp('v (rear_stiff_sw) [-]')
  steer_max [deg] : Subsystem
      mask Display: disp('v (steer_max) [deg]')
  steer_min [deg] : Subsystem
      mask Display: disp('v (steer_min) [deg]')
  steer_rate_max [deg/s] : Subsystem
      mask Display: disp('v (steer_rate_max) [deg/s]')
  steer_rate_min [deg/s] : Subsystem
      mask Display: disp('v (steer_rate_min) [deg/s]')
  steer_smooth_t [s] : Subsystem
      mask Display: disp('v (steer_smooth_t) [s]')
  target_aim_x [m] : Subsystem
      mask Display: disp('v (target_aim_x) [m]')
  tgt_a_max [m/s^2] : Subsystem
      mask Display: disp('v (tgt_a_max) [m/s^2]')
  tgt_acc_smooth_t [s] : Subsystem
      mask Display: disp('v (tgt_acc_smooth_t) [s]')
  tgt_ax_max [m/s^2] : Subsystem
      mask Display: disp('v (tgt_ax_max) [m/s^2]')
  tgt_ax_min [m/s^2] : Subsystem
      mask Display: disp('v (tgt_ax_min) [m/s^2]')
  tgt_ay_max [m/s^2] : Subsystem
      mask Display: disp('v (tgt_ay_max) [m/s^2]')
  tgt_v_max [m/s] : Subsystem
      mask Display: disp('v (tgt_v_max) [m/s]')
  tgt_v_min [m/s] : Subsystem
      mask Display: disp('v (tgt_v_min) [m/s]')
  use_simulink_sw [-] : Subsystem
      mask Display: disp('v (use_simulink_sw) [-]')
  v_comp_scale [-] : Subsystem
      mask Display: disp('v (v_comp_scale) [-]')
  v_path [m/s] : Subsystem
      mask Display: disp('desired velocity [m/s]')

== system Demo_veDYNA_cs/Vedyna_Vehicle/CPT_MDL/MDL_PAR/Engine/System Instance 1 ==
  ASR_Flag [-] : Subsystem
      mask Display: disp('ASR Flag [-]')
  ASR_Torque [Nm] : Subsystem
      mask Display: disp('ASR Torque [Nm]')
  MSR_Flag [-] : Subsystem
      mask Display: disp('MSR Flag [-]')
  MSR_Torque [Nm] : Subsystem
      mask Display: disp('MSR Torque [Nm]')

== system Demo_veDYNA_cs/Vedyna_Vehicle/CPT_MDL/MDL_PAR/GearCtrl/System Instance 1 ==
  Gear [-] : Subsystem
      mask Display: disp('Gear position [-]')
  UpShiftRequest [-1,1] : Subsystem
      mask Display: disp('Up shift request [-1,1]')

== system Demo_veDYNA_cs/Vedyna_Vehicle/CPT_MDL/MDL_PAR/ManLatCtrl/System Instance 1 ==
  Curvature [1/m] : Subsystem
      mask Display: disp('Curvature [1/m]')
  Steering [deg] : Subsystem
      mask Display: disp('Steering wheel angle [deg]')

== system Demo_veDYNA_cs/Vedyna_Vehicle/CPT_MDL/MDL_PAR/ManLongCtrl/System Instance 1 ==
  AccelerationY [m/s**2] : Subsystem
      mask Display: disp('Lateral acceleration [m/s**2]')
  Brake [%] : Subsystem
      mask Display: disp('Brake position [%]')
  EngineTorque [Nm] : Subsystem
      mask Display: disp('Engine torque [Nm]')
  Speed [km/h] : Subsystem
      mask Display: disp('Speed [km/h]')
  Throttle [%] : Subsystem
      mask Display: disp('Throttle position [%]')

== system Demo_veDYNA_cs/Vedyna_Vehicle/CPT_MDL/MDL_PAR/Tmeasy/System Instance 1 ==
  RoadMueScale [0..1] : Subsystem
      mask Display: disp('Road mue scaling factor [0..1]')

== system Demo_veDYNA_cs/Vedyna_Vehicle/CPT_MDL/MDL_PAR/Tmeasy/System Instance 2 ==
  RoadMueScale [0..1] : Subsystem
      mask Display: disp('Road mue scaling factor [0..1]')

== system Demo_veDYNA_cs/Vedyna_Vehicle/CPT_MDL/MDL_PAR/Tmeasy/System Instance 3 ==
  RoadMueScale [0..1] : Subsystem
      mask Display: disp('Road mue scaling factor [0..1]')

== system Demo_veDYNA_cs/Vedyna_Vehicle/CPT_MDL/MDL_PAR/Tmeasy/System Instance 4 ==
  RoadMueScale [0..1] : Subsystem
      mask Display: disp('Road mue scaling factor [0..1]')

== system Demo_veDYNA_cs/Vedyna_Vehicle/CPT_MDL/MDL_PAR/Tmeasy/System Instance 5 ==
  RoadMueScale [0..1] : Subsystem
      mask Display: disp('Road mue scaling factor [0..1]')

== system Demo_veDYNA_cs/Vedyna_Vehicle/CPT_MDL/MDL_PAR/Tmeasy/System Instance 6 ==
  RoadMueScale [0..1] : Subsystem
      mask Display: disp('Road mue scaling factor [0..1]')

== system Demo_veDYNA_cs/Vedyna_Vehicle/CPT_MDL/MDL_PAR/Tmeasy/System Instance 7 ==
  RoadMueScale [0..1] : Subsystem
      mask Display: disp('Road mue scaling factor [0..1]')

== system Demo_veDYNA_cs/Vedyna_Vehicle/CPT_MDL/MDL_PAR/Tmeasy/System Instance 8 ==
  RoadMueScale [0..1] : Subsystem
      mask Display: disp('Road mue scaling factor [0..1]')

== system Demo_veDYNA_cs/Vedyna_Vehicle/CPT_MDL/MDL_PAR/Wheel/System Instance 1 ==
  pbrm [N/m**2] : Subsystem
      mask Display: disp('Wheel cylinder brake pressure [N/m**2]')

== system Demo_veDYNA_cs/Vedyna_Vehicle/CPT_MDL/MDL_PAR/Wheel/System Instance 2 ==
  pbrm [N/m**2] : Subsystem
      mask Display: disp('Wheel cylinder brake pressure [N/m**2]')

== system Demo_veDYNA_cs/Vedyna_Vehicle/CPT_MDL/MDL_PAR/Wheel/System Instance 3 ==
  pbrm [N/m**2] : Subsystem
      mask Display: disp('Wheel cylinder brake pressure [N/m**2]')

== system Demo_veDYNA_cs/Vedyna_Vehicle/CPT_MDL/MDL_PAR/Wheel/System Instance 4 ==
  pbrm [N/m**2] : Subsystem
      mask Display: disp('Wheel cylinder brake pressure [N/m**2]')

== system Demo_veDYNA_cs/Vedyna_Vehicle/CPT_MDL/MDL_PAR/Wheel/System Instance 5 ==
  pbrm [N/m**2] : Subsystem
      mask Display: disp('Wheel cylinder brake pressure [N/m**2]')

== system Demo_veDYNA_cs/Vedyna_Vehicle/CPT_MDL/MDL_PAR/Wheel/System Instance 6 ==
  pbrm [N/m**2] : Subsystem
      mask Display: disp('Wheel cylinder brake pressure [N/m**2]')

== system Demo_veDYNA_cs/Vedyna_Vehicle/CPT_MDL/MDL_PAR/Wheel/System Instance 7 ==
  pbrm [N/m**2] : Subsystem
      mask Display: disp('Wheel cylinder brake pressure [N/m**2]')

== system Demo_veDYNA_cs/Vedyna_Vehicle/CPT_MDL/MDL_PAR/Wheel/System Instance 8 ==
  pbrm [N/m**2] : Subsystem
      mask Display: disp('Wheel cylinder brake pressure [N/m**2]')

== system Demo_veDYNA_cs/Vedyna_Vehicle/CPT_MDL/MDL_SW/BrkHyd/System Instance 1 ==
  HCI [1,..,n] : Subsystem
      mask Display: disp('HCI switch [1,..,n]')
  pbrmaster [1,..,4] : Subsystem
      mask Display: disp('Input switch: value(1), table(2), io(3), other(4) [1,..,4]')

== system Demo_veDYNA_cs/Vedyna_Vehicle/CPT_MDL/MDL_SW/Chassis/System Instance 1 ==
  HCI [1,..,n] : Subsystem
      mask Display: disp('HCI switch [1,..,n]')

== system Demo_veDYNA_cs/Vedyna_Vehicle/CPT_MDL/MDL_SW/ClutchCtrl/System Instance 1 ==
  Clutch [1,..,4] : Subsystem
      mask Display: disp('Input switch: value(1), table(2), io(3), other(4) [1,..,4]')
  ClutchMode [0,1] : Subsystem
      mask Display: disp('Input switch: internal(0), external(1) [0,1]')
  HCI [1,..,n] : Subsystem
      mask Display: disp('HCI switch [1,..,n]')

== system Demo_veDYNA_cs/Vedyna_Vehicle/CPT_MDL/MDL_SW/Contact/System Instance 1 ==
  RoadZ [1,..,4] : Subsystem
      mask Display: disp('Input switch: value(1), table(2), io(3), other(4) [1,..,4]')

== system Demo_veDYNA_cs/Vedyna_Vehicle/CPT_MDL/MDL_SW/Contact/System Instance 2 ==
  RoadZ [1,..,4] : Subsystem
      mask Display: disp('Input switch: value(1), table(2), io(3), other(4) [1,..,4]')

== system Demo_veDYNA_cs/Vedyna_Vehicle/CPT_MDL/MDL_SW/Contact/System Instance 3 ==
  RoadZ [1,..,4] : Subsystem
      mask Display: disp('Input switch: value(1), table(2), io(3), other(4) [1,..,4]')

== system Demo_veDYNA_cs/Vedyna_Vehicle/CPT_MDL/MDL_SW/Contact/System Instance 4 ==
  RoadZ [1,..,4] : Subsystem
      mask Display: disp('Input switch: value(1), table(2), io(3), other(4) [1,..,4]')

== system Demo_veDYNA_cs/Vedyna_Vehicle/CPT_MDL/MDL_SW/Contact/System Instance 5 ==
  RoadZ [1,..,4] : Subsystem
      mask Display: disp('Input switch: value(1), table(2), io(3), other(4) [1,..,4]')

== system Demo_veDYNA_cs/Vedyna_Vehicle/CPT_MDL/MDL_SW/Contact/System Instance 6 ==
  RoadZ [1,..,4] : Subsystem
      mask Display: disp('Input switch: value(1), table(2), io(3), other(4) [1,..,4]')

== system Demo_veDYNA_cs/Vedyna_Vehicle/CPT_MDL/MDL_SW/Contact/System Instance 7 ==
  RoadZ [1,..,4] : Subsystem
      mask Display: disp('Input switch: value(1), table(2), io(3), other(4) [1,..,4]')

== system Demo_veDYNA_cs/Vedyna_Vehicle/CPT_MDL/MDL_SW/Contact/System Instance 8 ==
  RoadZ [1,..,4] : Subsystem
      mask Display: disp('Input switch: value(1), table(2), io(3), other(4) [1,..,4]')

== system Demo_veDYNA_cs/Vedyna_Vehicle/CPT_MDL/MDL_SW/Driveline/System Instance 1 ==
  HCI [1,..,n] : Subsystem
      mask Display: disp('HCI switch [1,..,n]')

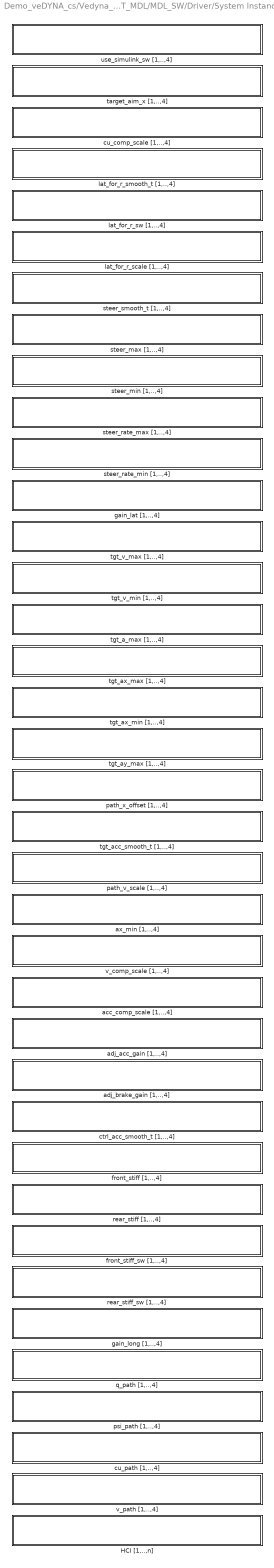
== system Demo_veDYNA_cs/Vedyna_Vehicle/CPT_MDL/MDL_SW/Driver/System Instance 1 ==
  HCI [1,..,n] : Subsystem
      mask Display: disp('HCI switch [1,..,n]')
  acc_comp_scale [1,..,4] : Subsystem
      mask Display: disp('Input switch: value(1), table(2), io(3), other(4) [1,..,4]')
  adj_acc_gain [1,..,4] : Subsystem
      mask Display: disp('Input switch: value(1), table(2), io(3), other(4) [1,..,4]')
  adj_brake_gain [1,..,4] : Subsystem
      mask Display: disp('Input switch: value(1), table(2), io(3), other(4) [1,..,4]')
  ax_min [1,..,4] : Subsystem
      mask Display: disp('Input switch: value(1), table(2), io(3), other(4) [1,..,4]')
  ctrl_acc_smooth_t [1,..,4] : Subsystem
      mask Display: disp('Input switch: value(1), table(2), io(3), other(4) [1,..,4]')
  cu_comp_scale [1,..,4] : Subsystem
      mask Display: disp('Input switch: value(1), table(2), io(3), other(4) [1,..,4]')
  cu_path [1,..,4] : Subsystem
      mask Display: disp('Input switch: value(1), table(2), io(3), other(4) [1,..,4]')
  front_stiff [1,..,4] : Subsystem
      mask Display: disp('Input switch: value(1), table(2), io(3), other(4) [1,..,4]')
  front_stiff_sw [1,..,4] : Subsystem
      mask Display: disp('Input switch: value(1), table(2), io(3), other(4) [1,..,4]')
  gain_lat [1,..,4] : Subsystem
      mask Display: disp('Input switch: value(1), table(2), io(3), other(4) [1,..,4]')
  gain_long [1,..,4] : Subsystem
      mask Display: disp('Input switch: value(1), table(2), io(3), other(4) [1,..,4]')
  lat_for_r_scale [1,..,4] : Subsystem
      mask Display: disp('Input switch: value(1), table(2), io(3), other(4) [1,..,4]')
  lat_for_r_smooth_t [1,..,4] : Subsystem
      mask Display: disp('Input switch: value(1), table(2), io(3), other(4) [1,..,4]')
  lat_for_r_sw [1,..,4] : Subsystem
      mask Display: disp('Input switch: value(1), table(2), io(3), other(4) [1,..,4]')
  path_v_scale [1,..,4] : Subsystem
      mask Display: disp('Input switch: value(1), table(2), io(3), other(4) [1,..,4]')
  path_x_offset [1,..,4] : Subsystem
      mask Display: disp('Input switch: value(1), table(2), io(3), other(4) [1,..,4]')
  psi_path [1,..,4] : Subsystem
      mask Display: disp('Input switch: value(1), table(2), io(3), other(4) [1,..,4]')
  q_path [1,..,4] : Subsystem
      mask Display: disp('Input switch: value(1), table(2), io(3), other(4) [1,..,4]')
  rear_stiff [1,..,4] : Subsystem
      mask Display: disp('Input switch: value(1), table(2), io(3), other(4) [1,..,4]')
  rear_stiff_sw [1,..,4] : Subsystem
      mask Display: disp('Input switch: value(1), table(2), io(3), other(4) [1,..,4]')
  steer_max [1,..,4] : Subsystem
      mask Display: disp('Input switch: value(1), table(2), io(3), other(4) [1,..,4]')
  steer_min [1,..,4] : Subsystem
      mask Display: disp('Input switch: value(1), table(2), io(3), other(4) [1,..,4]')
  steer_rate_max [1,..,4] : Subsystem
      mask Display: disp('Input switch: value(1), table(2), io(3), other(4) [1,..,4]')
  steer_rate_min [1,..,4] : Subsystem
      mask Display: disp('Input switch: value(1), table(2), io(3), other(4) [1,..,4]')
  steer_smooth_t [1,..,4] : Subsystem
      mask Display: disp('Input switch: value(1), table(2), io(3), other(4) [1,..,4]')
  target_aim_x [1,..,4] : Subsystem
      mask Display: disp('Input switch: value(1), table(2), io(3), other(4) [1,..,4]')
  tgt_a_max [1,..,4] : Subsystem
      mask Display: disp('Input switch: value(1), table(2), io(3), other(4) [1,..,4]')
  tgt_acc_smooth_t [1,..,4] : Subsystem
      mask Display: disp('Input switch: value(1), table(2), io(3), other(4) [1,..,4]')
  tgt_ax_max [1,..,4] : Subsystem
      mask Display: disp('Input switch: value(1), table(2), io(3), other(4) [1,..,4]')
  tgt_ax_min [1,..,4] : Subsystem
      mask Display: disp('Input switch: value(1), table(2), io(3), other(4) [1,..,4]')
  tgt_ay_max [1,..,4] : Subsystem
      mask Display: disp('Input switch: value(1), table(2), io(3), other(4) [1,..,4]')
  tgt_v_max [1,..,4] : Subsystem
      mask Display: disp('Input switch: value(1), table(2), io(3), other(4) [1,..,4]')
  tgt_v_min [1,..,4] : Subsystem
      mask Display: disp('Input switch: value(1), table(2), io(3), other(4) [1,..,4]')
  use_simulink_sw [1,..,4] : Subsystem
      mask Display: disp('Input switch: value(1), table(2), io(3), other(4) [1,..,4]')
  v_comp_scale [1,..,4] : Subsystem
      mask Display: disp('Input switch: value(1), table(2), io(3), other(4) [1,..,4]')
  v_path [1,..,4] : Subsystem
      mask Display: disp('Input switch: value(1), table(2), io(3), other(4) [1,..,4]')

== system Demo_veDYNA_cs/Vedyna_Vehicle/CPT_MDL/MDL_SW/Engine/System Instance 1 ==
  ASR_Flag [1,..,4] : Subsystem
      mask Display: disp('Input switch: value(1), table(2), io(3), other(4) [1,..,4]')
  ASR_Torque [1,..,4] : Subsystem
      mask Display: disp('Input switch: value(1), table(2), io(3), other(4) [1,..,4]')
  HCI [1,..,n] : Subsystem
      mask Display: disp('[Generated]')
  MSR_Flag [1,..,4] : Subsystem
      mask Display: disp('Input switch: value(1), table(2), io(3), other(4) [1,..,4]')
  MSR_Torque [1,..,4] : Subsystem
      mask Display: disp('Input switch: value(1), table(2), io(3), other(4) [1,..,4]')
